simulink model "F16_FinalDemo"  (R2024b)
settings: Solver=ode4  StartTime=0.0  StopTime=30  FixedStep=0.01  RelTol=1e-3
undefined symbols (not defined in the file): fb_gain, fi_flag_Simulink, init_dlef, init_u_base, K_long, x_ref_long
settings Model: Creator=nefelibata  LastModifiedBy=nefelibata
settings DataIOCC: SaveState=on

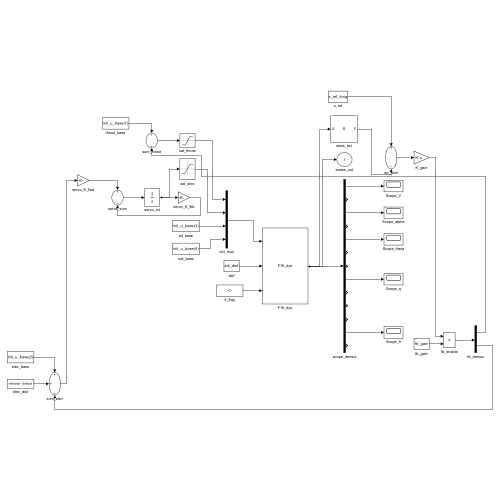
[thumbnail: Simulink's stored preview of the top-level diagram]
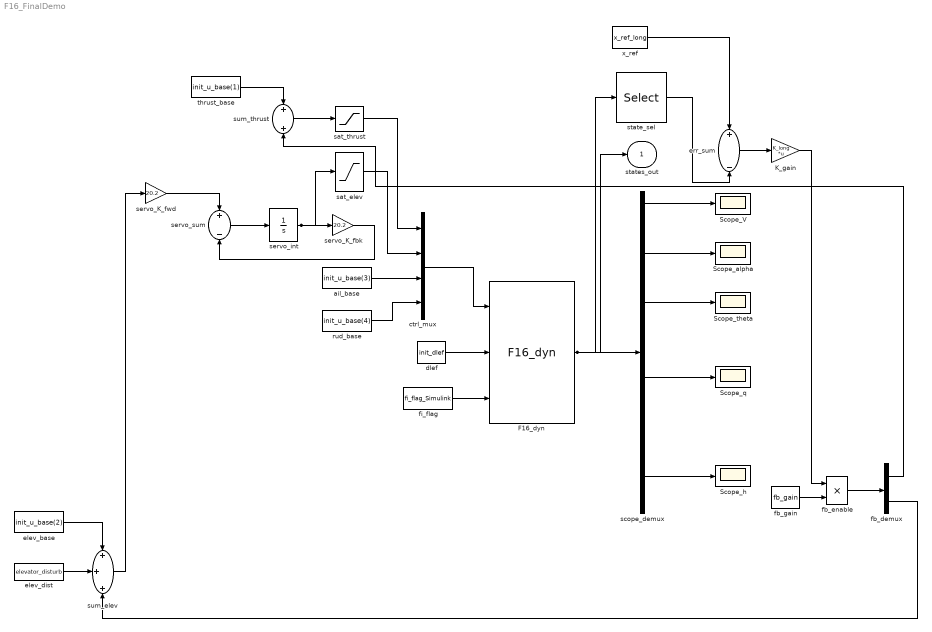
== system F16_FinalDemo ==
  F16_dyn : S-Function  FunctionName=F16_dyn  Parameters=init_x  SFunctionDeploymentMode=off  EnableBusSupport=off
  K_gain : Gain  Gain=K_long  Multiplication=Matrix(K*u)
  Scope_V : Scope
  Scope_alpha : Scope
  Scope_h : Scope
  Scope_q : Scope
  Scope_theta : Scope
  ail_base : Constant  Value=init_u_base(3)
  ctrl_mux : Mux
  dlef : Constant  Value=init_dlef
  elev_base : Constant  Value=init_u_base(2)
  elev_dist : FromWorkspace  VariableName=elevator_disturb  SampleTime=0.01  OutputAfterFinalValue=Setting to zero
  err_sum : Sum  Inputs=+-
  fb_demux : Demux  Outputs=2
  fb_enable : Product  Inputs=**
  fb_gain : Constant  Value=fb_gain
  fi_flag : Constant  Value=fi_flag_Simulink
  rud_base : Constant  Value=init_u_base(4)
  sat_elev : Saturate  UpperLimit=0.44  LowerLimit=-0.44
  sat_thrust : Saturate  UpperLimit=1  LowerLimit=0
  scope_demux : Demux  Outputs=13
  servo_K_fbk : Gain  Gain=20.2
  servo_K_fwd : Gain  Gain=20.2
  servo_int : Integrator  InitialCondition=-0.02672333065541166
  servo_sum : Sum  Inputs=+-
  state_sel : Selector  InputPortWidth=13  IndexOptions=Index vector (dialog)  Indices=[1,3,5,8,13]  OutputSizes=1
  sum_elev : Sum  Inputs=+++
  sum_thrust : Sum
  thrust_base : Constant  Value=init_u_base(1)
  x_ref : Constant  Value=x_ref_long
  states_out : Outport
  wires:
  sum_thrust/1 -> sat_thrust/1
  ail_base/1 -> ctrl_mux/3
  thrust_base/1 -> sum_thrust/1
  elev_base/1 -> sum_elev/1
  dlef/1 -> F16_dyn/2
  servo_K_fwd/1 -> servo_sum/1
  servo_sum/1 -> servo_int/1
  elev_dist/1 -> sum_elev/2
  sum_elev/1 -> servo_K_fwd/1
  servo_int/1 -> servo_K_fbk/1, sat_elev/1
  sat_thrust/1 -> ctrl_mux/1
  sat_elev/1 -> ctrl_mux/2
  servo_K_fbk/1 -> servo_sum/2
  fb_enable/1 -> fb_demux/1
  K_gain/1 -> fb_enable/1
  rud_base/1 -> ctrl_mux/4
  ctrl_mux/1 -> F16_dyn/1
  fi_flag/1 -> F16_dyn/3
  err_sum/1 -> K_gain/1
  F16_dyn/1 -> state_sel/1, states_out/1, scope_demux/1
  x_ref/1 -> err_sum/1
  scope_demux/3 -> Scope_alpha/1
  state_sel/1 -> err_sum/2
  fb_demux/2 -> sum_elev/3
  scope_demux/1 -> Scope_V/1
  scope_demux/5 -> Scope_theta/1
  scope_demux/8 -> Scope_q/1
  scope_demux/12 -> Scope_h/1
  fb_demux/1 -> sum_thrust/2
  fb_gain/1 -> fb_enable/2
